simulink model "sf_for"  (Simulink 7.6)
settings: Solver=FixedStepDiscrete  StartTime=0.0  StopTime=1  FixedStep=1  RelTol=1e-3
settings Model: Creator=The MathWorks Inc.  CovMetricSettings=dcmtr  ExtModeAutoUpdateStatusClock=off
settings DataIOCC: SignalLoggingName=sigsOut
settings OptimizationCC: InlineInvariantSignals=on  InitFltsAndDblsToZero=on  EfficientMapNaN2IntZero=off  BufferReusableBoundary=off
settings DebuggingCC: SaveWithParameterizedLinksMsg=none  SignalResolutionControl=TryResolveAllWithWarning  SolverPrmCheckMsg=none  MultiTaskDSMMsg=warning  MultiTaskCondExecSysMsg=none  StrictBusMsg=None
settings HardwareCC: TargetUnknown=on
settings SFSimCC: SimParseCustomCode=off
settings RTWCC: IncludeERTFirstTime=on
settings GRTTargetCC: TargetFcnLib=ansi_tfl_tmw.mat

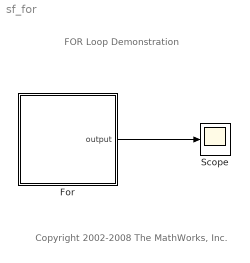
== system sf_for ==
  note: FOR Loop Demonstration
  note: Copyright 2002-2008 The MathWorks, Inc.
  For : Stateflow chart  TreatAsAtomicUnit=on
  Scope : Scope
      settings: TimeRange=1  YMin=0  YMax=20
  wires:
  For/1(output) -> Scope/1

== stateflow chart For ==
  note: Equivalent C-Code:
      | for(i=0;i <10;i++)
      | {
      |      output[i] = 2 * i;
      | }
  (default) -> (junction 4) : { i = 0;}
  (junction 4) -> (junction 5)
  (junction 5) -> (junction 6) [order 2]
  (junction 5) -> (junction 4) [order 1] : [i < 10]{ output[i] = 2 * i; i++;}
  data: i local int32; output output int32 size=[10]
